simulink model "Solution3_RFReceiverWithXdipole"  (R2024b)
settings: Solver=VariableStepAuto  StartTime=0.0  StopTime=inf  RelTol=1e-3  EnableMultiTasking=on
PreLoadFcn:
  | % Baseband parameters
  | bitRate = 250e3;
  | spf = 4;  % samples per frame
  | bps = 4;  % bits per ZigBee symbol
  | sps = 16;  % samples per OQPSK symbol
  | cps = 32;  % chips per ZigBee symbol
  | chipRate = bitRate * cps / bps;
  | 
  | % RF parameters
  | carrierFreqs = [2.45 2.5]*1e9;  % Hz
  | harmonicOrder = [1 3];
  | oversampling = 4;  % reduce RF simulation step size to simulate interferer
  | load('XdipoleAntenna.mat')
undefined symbols (not defined in the file): rational, S, SampTime, sparameters
libraries: simrfV2elements x7, commdigbbndpm3 x3, simrfV2util1 x3, commrandsrc3 x2, dspmathops x2, dspsigops x2, dspstat3 x2, matrix_library x2, simulink x1, commrfcorlib x1, commrflib2 x1, commsink2 x1
Description:
  | Top-Down Design of Spread Spectrum Receiver for ZigBee
settings Model: Creator=The MathWorks, Inc.  LastModifiedBy=maxnolan
settings SolverCC: AlgebraicLoopSolver=TrustRegion  MinimalZcImpactIntegration=on  MaxZcPerStep=1
settings DataIOCC: LimitDataPoints=on  SaveFormat=Array  SaveOutput=off  SignalLogging=off  DSMLogging=off  SaveTime=off  ReturnWorkspaceOutputs=off
settings OptimizationCC: ReuseModelBlockBuffer=off  ExpressionDepthLimit=2147483647  LifeSpan=inf
settings DebuggingCC: ConsistencyChecking=warning  UnderspecifiedInitializationDetection=Classic  MergeDetectMultiDrivingBlocksExec=none  TimeAdjustmentMsg=warning  MaxConsecutiveZCsMsg=warning  SolverPrmCheckMsg=warning  FcnCallInpInsideContextMsg=warning  UnconnectedInputMsg=warning  UnconnectedOutputMsg=warning  UnconnectedLineMsg=warning  StateNameClashWarn=warning  SFUnexpectedBacktrackingDiag=warning  SFNoUnconditionalDefaultTransitionDiag=warning  SFExecutionAtInitializationDiag=none  ArithmeticOperatorsInVariantConditions=warning
settings HardwareCC: ProdBitPerPointer=32  ProdBitPerSizeT=32  ProdBitPerPtrDiffT=32  ProdLargestAtomicFloat=None  ProdIntDivRoundTo=Undefined  ProdEndianess=Unspecified  ProdWordSize=32  ProdHWDeviceType=32-bit Generic
settings ModelReferenceCC: EnableRefExpFcnMdlSchedulingChecks=on  PropagateSignalLabelsOutOfModel=off
settings SFSimCC: SimUseLocalCustomCode=off
settings RTWCC: RTWUseLocalCustomCode=off  BuildConfiguration=Faster Runs  GPUComputeCapability=3.5  DLArmComputeVersion=19.05
settings CodeAppCC: StateflowObjectComments=on
settings GRTTargetCC: TargetLangStandard=C89/C90 (ANSI)  CombineOutputUpdateFcns=off  GRTInterface=on
settings ConfigComp: CovMetricSettings=dw  CovSaveCumulativeToWorkspaceVar=on  CovSaveSingleToWorkspaceVar=on  CovExternalEMLEnable=off  CovSFcnEnable=off
settings SimscapeCC: SimscapeNormalizeSystem=off  SimscapeNominalValues="[{\"value\":\"10\",\"unit\":\"V\"},{\"value\":\"1\",\"unit\":\"A\"},{\"value\":\"10\",\"unit\":\"N*m\"},{\"value\":\"10\",\"unit\":\"bar\"},{\"value\":\"100\",\"unit\":\"kJ/kg\"},{\"value\":\"1\",\"unit\":\"kW\"},{\"value\":\"300\",\"unit\":\"K\"},{\"value\":\"100\",\"unit\":\"cm^3/s\"},{\"value\":\"1\",\"unit\":\"kN\"},{\"value\":\"1\",\"unit\":\"g/cm^3\"},{\"value\":\"1\",\"unit\":\"l\"},{\"value\":\"1\",\"unit\":\"cm^2\"},{\"value\":\"60\",\"unit\":\"Hz\"}]"
settings ConfigurationSet: Description=SimMechanics 2G

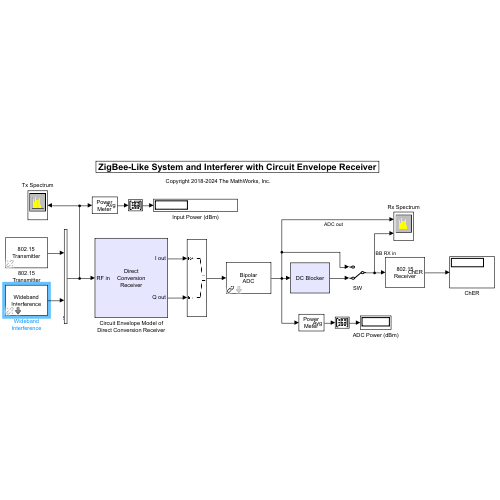
[thumbnail: Simulink's stored preview of the top-level diagram]
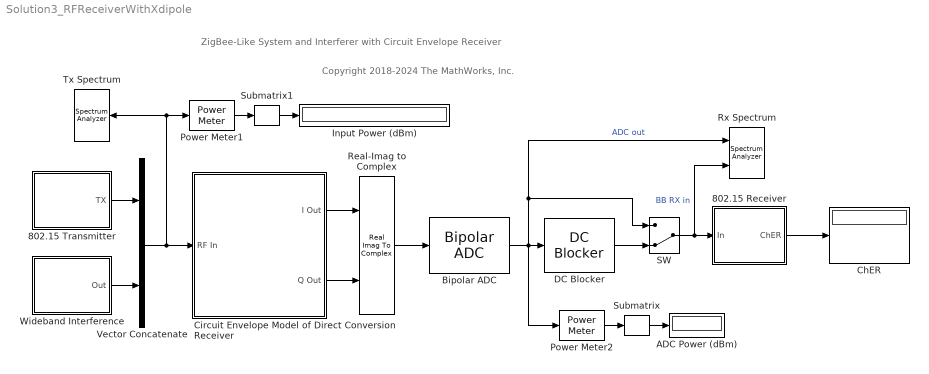
== system Solution3_RFReceiverWithXdipole ==
  note: ZigBee-Like System and Interferer with Circuit Envelope Receiver
  note: Copyright 2018-2024 The MathWorks, Inc.
  802.15 Transmitter : Subsystem  AncestorBlock=TopDownRFReceiverDesignLib/802.15 Transmitter
      mask Display: disp('802.15\nTransmitter')
  802.15 Receiver : Subsystem
      mask Display:
      | disp('802.15\nReceiver')
      | port_label('output', 1, 'ChER')
  ADC Power (dBm) : Display
  Bipolar ADC : TopDownRFReceiverDesignLib/Bipolar ADC  FS_V=sqrt(10^((0-30)/10))  N=10
      settings: LibrarySourceBlock=commdemoslib/Bipolar ADC
  ChER : Display
  Circuit Envelope Model of Direct Conversion Receiver : Subsystem
      mask Display:
      | disp('Direct\nConversion\nReceiver')
      | port_label('input', 1, 'RF in')
      | port_label('output', 1, 'I out')
      | port_label('output', 2, 'Q out')
  DC Blocker : dspsigops/DC Blocker  Algorithm=IIR  NormalizedBandwidth=0.001  Length=64  Order=16  SimulateUsing=Interpreted execution
  Input Power (dBm) : Display
  Power Meter1 : dspstat3/Power Meter  Measurement=Average power  ReferenceLoad=1  OutputPowerUnits=dBm  WindowLength=1024  OverlapLength=1023  AllowArbitraryInputLength=off  ComputeCCDF=off  PowerRange=50  PowerResolution=0.1  CCDFOutput=Relative power (dB above average power)  ProbabilityVector=[ 10; 1; 0.1; 0.01; 0.001; 0.0001 ]  RelativePowerVector=[ 0; 3; 6; 9; 12 ]  ResetPort=off  SimulateUsing=Code generation
      settings: LibrarySourceBlock=commutil2/Power Meter
  Power Meter2 : dspstat3/Power Meter  Measurement=Average power  ReferenceLoad=1  OutputPowerUnits=dBm  WindowLength=1024  OverlapLength=1023  AllowArbitraryInputLength=off  ComputeCCDF=off  PowerRange=50  PowerResolution=0.1  CCDFOutput=Relative power (dB above average power)  ProbabilityVector=[ 10; 1; 0.1; 0.01; 0.001; 0.0001 ]  RelativePowerVector=[ 0; 3; 6; 9; 12 ]  ResetPort=off  SimulateUsing=Code generation
      settings: LibrarySourceBlock=commutil2/Power Meter
  Real-Imag to Complex : RealImagToComplex
  Rx Spectrum : SpectrumAnalyzer  NumInputPorts=2  WindowPosition=[540.000000,122.000000,475.000000,318.000000,]  ScopeFrameLocation=window  Method=Welch  SampleRate=16000000  AxesScaling=Manual  FrequencyResolutionMethod=Window length  RBWSource=Property  RBW=46921.92192  FFTLength=128  Span=32000000  StartFrequency=-16000000  StopFrequency=16000000  AveragingMethod=Running  SpectralAverages=16  YLabel=Power  YLimits=[-75.64216798,-32.23249525]  ShowLegend=on  AllowFFTLengthLessThanSamplesPerUpdate=on  SegLen=1024
  SW : ManualSwitch  CurrentSetting=0
  Submatrix : matrix_library/Submatrix  RowSpan=One row  RowStartMode=Last  RowStartIndex=1  RowEndMode=Last  RowEndIndex=1  ColSpan=One column  ColStartMode=Last  ColStartIndex=1  ColEndMode=Last  ColEndIndex=1
  Submatrix1 : matrix_library/Submatrix  RowSpan=One row  RowStartMode=Last  RowStartIndex=1  RowEndMode=Last  RowEndIndex=1  ColSpan=Range of columns  ColStartMode=Offset from last  ColStartIndex=1  ColEndMode=Last  ColEndIndex=1
  Tx Spectrum : SpectrumAnalyzer  WindowPosition=[21.000000,122.000000,520.000000,320.000000,]  ScopeFrameLocation=window  Method=Welch  SampleRate=16000000  AxesScaling=Manual  FrequencyResolutionMethod=Window length  RBWSource=Property  RBW=46921.92192  FFTLength=128  Span=16000000  StartFrequency=-16000000  StopFrequency=16000000  AveragingMethod=Running  SpectralAverages=16  FrequencyOffset=carrierFreqs  YLabel=Power  YLimits=[-211.4024859,-30.13598267]  ShowLegend=on  AllowFFTLengthLessThanSamplesPerUpdate=on  SegLen=1024
  Vector Concatenate : Concatenate  Mode=Multidimensional array  ConcatenateDimension=2
  Wideband Interference : Subsystem  AncestorBlock=TopDownRFReceiverDesignLib/Wideband Interference  mask{Pout=-30}
      mask prompts: Pout "Output power (dBm)"
      mask Display: disp('Wideband\nInterference')
  wires:
  802.15 Receiver/1(ChER) -> ChER/1
  Circuit Envelope Model of Direct Conversion Receiver/1(I Out) -> Real-Imag to Complex/1
  Circuit Envelope Model of Direct Conversion Receiver/2(Q Out) -> Real-Imag to Complex/2
  Bipolar ADC/1 -> Power Meter2/1, DC Blocker/1, SW/1, Rx Spectrum/1  "ADC out"
  Vector Concatenate/1 -> Circuit Envelope Model of Direct Conversion Receiver/1(RF In), Tx Spectrum/1, Power Meter1/1
  Power Meter1/1 -> Submatrix1/1
  802.15 Transmitter/1(TX) -> Vector Concatenate/1
  Power Meter2/1 -> Submatrix/1
  DC Blocker/1 -> SW/2
  SW/1 -> Rx Spectrum/2, 802.15 Receiver/1(In)  "BB RX in"
  Submatrix/1 -> ADC Power (dBm)/1
  Submatrix1/1 -> Input Power (dBm)/1
  Wideband Interference/1(Out) -> Vector Concatenate/2
  Real-Imag to Complex/1 -> Bipolar ADC/1

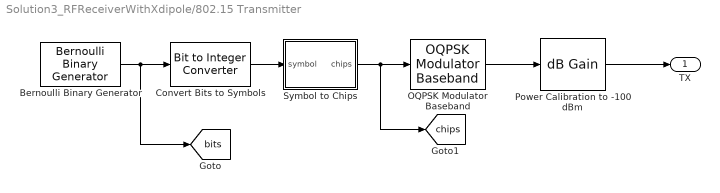
== system Solution3_RFReceiverWithXdipole/802.15 Transmitter ==
  Bernoulli Binary Generator : commrandsrc3/Bernoulli Binary Generator  ProbabilityOfZero=0.5  SeedSource=Parameter  Seed=73  SampleTime=1/bitRate  SamplesPerFrame=spf  OutputDataType=double  SimulateUsing=Interpreted execution
  Convert Bits to Symbols : simulink/Logic and Bit Operations/Bit to Integer Converter  nbits=4  bitOrder=MSB first  signedOutputValues=Unsigned  outDtype=Inherit via internal rule  outDtypeSigned=Inherit via internal rule
      settings: LibrarySourceBlock=|
      | commutil2/Bit to Integer
      | Converter
  OQPSK Modulator Baseband : commdigbbndpm3/OQPSK Modulator Baseband  InType=Bit  Ph=0  Mapping=Gray  pulseShape=Half sine  num=[0.7071, 0.7071]  rolloff=0.2  filterSpan=10  sps=sps  RateOptions=Enforce single-rate processing  outDtype=double
  Power Calibration to -100 dBm : dspmathops/dB Gain  dB="-130  % power of preceding block is 1 W"  intype=Amplitude
  Symbol to Chips : MATLAB Function  TreatAsAtomicUnit=on
  TX : Outport  VectorParamsAs1DForOutWhenUnconnected=off
  tag scope: bits=global, chips=global
  wires:
  Bernoulli Binary Generator/1 -> [bits], Convert Bits to Symbols/1
  Symbol to Chips/1(chips) -> [chips], OQPSK Modulator Baseband/1
  Convert Bits to Symbols/1 -> Symbol to Chips/1(symbol)
  OQPSK Modulator Baseband/1 -> Power Calibration to -100 dBm/1
  Power Calibration to -100 dBm/1 -> TX/1

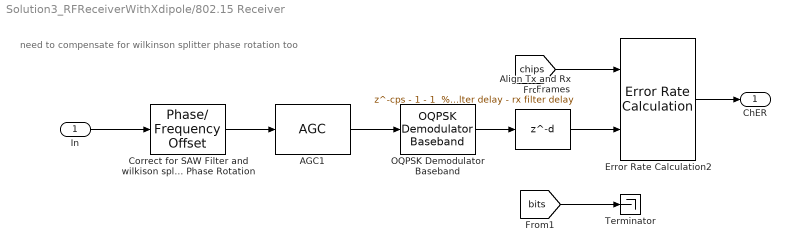
== system Solution3_RFReceiverWithXdipole/802.15 Receiver ==
  note: need to compensate for wilkinson splitter phase rotation too
  In : Inport
  AGC1 : commrfcorlib/AGC  LegacyMode=off  DetectorMethod=Rectifier  LoopMethod=Linear  UpdatePeriod=100  StepSize=0.1  AdaptationStepSize=0.01  DesiredOutputPower=1  AveragingLength=100  MaximumGain=30  MaxPowerGain=200  GainOutputPort=off  InputPowerOutputPort=off  SimulateUsing=Interpreted execution
  Align Tx and Rx Frames : Delay  DelayLength="cps - 1 - 1  % chips/sym - tx filter delay - rx filter delay"  InputProcessing=Columns as channels (frame based)
  Correct for SAW Filter and wilkison splitter Phase Rotation : commrflib2/Phase// Frequency Offset  phaseOffset=115-90  freqPort=off  freqOffset=0
  Error Rate Calculation2 : commsink2/Error Rate Calculation  N="32  % 1 frame of chips"  st_delay=2e3  cp_mode=Entire frame  subframe=[]  PMode=Port  WsName=ErrorVec  RsMode2=off  stop=on  numErr=1e3  maxBits=1e7
  OQPSK Demodulator Baseband : commdigbbndpm3/OQPSK Demodulator Baseband  OutType=Bit  Ph=0  Mapping=Gray  pulseShape=Half sine  num=[0.7071, 0.7071]  rolloff=0.2  filterSpan=10  sps=sps  RateOptions=Enforce single-rate processing  outDtype2=double
  Terminator : Terminator
  ChER : Outport  VectorParamsAs1DForOutWhenUnconnected=off
  wires:
  Correct for SAW Filter and wilkison splitter Phase Rotation/1 -> AGC1/1
  Error Rate Calculation2/1 -> ChER/1
  [chips] -> Error Rate Calculation2/1
  In/1 -> Correct for SAW Filter and wilkison splitter Phase Rotation/1
  Align Tx and Rx Frames/1 -> Error Rate Calculation2/2
  OQPSK Demodulator Baseband/1 -> Align Tx and Rx Frames/1
  AGC1/1 -> OQPSK Demodulator Baseband/1
  [bits] -> Terminator/1

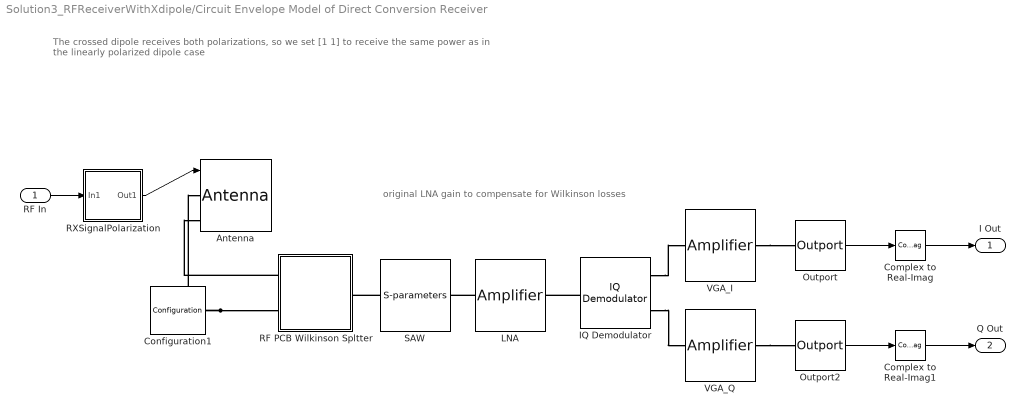
== system Solution3_RFReceiverWithXdipole/Circuit Envelope Model of Direct Conversion Receiver ==
  note: The crossed dipole receives both polarizations,
      | so we set [1 1] to receive the same power as in the linearly polarized dipole case
  note: original LNA gain to compensate for Wilkinson losses
  RF In : Inport
  Antenna : simrfV2elements/Antenna  CacheLevel=0  AntennaSource=Antenna object  PrevAppliedAntSource=Antenna object  Gr=0 dBi  Zin=50  AntennaObj=Xdipole  InputIncWave=on  OutputRadWave=off  CarrierFreqInc=carrierFreqs Hz  rArr=[0 0] deg  CarrierFreqRad=2.1 GHz  rDep=[0 0] deg  AddNoise=on  InternalGrounding=on  SparamRepresentationImp=Time domain  FitTolImp=-40  AutoImpulseLengthImp=on  ImpulseLengthImp=1e-10 s
  Complex to Real-Imag : ComplexToRealImag  Output=Real
  Complex to Real-Imag1 : ComplexToRealImag  Output=Real
  Configuration1 : simrfV2util1/Configuration  AutoFreq=off  Tones=carrierFreqs Hz  Harmonics=harmonicOrder  NormalizeCarrierPower=on  SolverType=Auto  UseCCode=on  StepSize=1/(2*chipRate*oversampling) s  AddNoise=on  defaultRNG=off  Seed=0  Temperature=290.0 K  SolverDelFlag=0  AbsTol=1e-6  RelTol=1e-3  MaxIter=10  ErrorEstimationType=2-norm over all variables  EnableInterpFilter=off  HiddenFIRfilterControllerParam=off  SmallSignalApprox=off  AllSimFreqs=on  SimFreqs=[] Hz  SimFreqsInternal=[]  SamplesPerFrame=cps * sps / 2
  "IQ Demodulator " : simrfV2systems/IQ Demodulator  classname=iqdemod  Source_linear_gain=Available power gain  linear_gain=-7 dB  Poly_Coeffs=[0 1]  LOFreq=2.45e9 Hz  Zin=50  Zout=50  AddIRFilter=off  AddCSFilters=on  InternalGrounding=on  ForceNextInit=off  Source_Poly=Even and odd order  IPType=Input  IP2=55 dBm  IP3=inf dBm  P1dB=inf dBm  Psat=inf dBm  Gcomp=inf dBm  NF=10  GainMismatch=0 dB  PhaseMismatch=0 deg  Isolation=105 dB  AddPhaseNoise=on  PhaseNoiseOffset=[0.2 1 2 3 7]*1e6  PhaseNoiseLevel=[-70 -80 -95 -110 -120]  AutoImpulseLengthPN=on  ImpulseLengthPN=5e-6  ImpulseLength_unitPN=s  DesignMethodIR=Ideal  ResponseTypeIR=Highpass  ImplementationIR=LC Tee  ImplementationIdealIR=Constant per carrier  ImplementationRationalIR=Transfer function  UseFilterOrderIR=on  FilterOrderIR=3  PassFreq_lpIR=1  PassFreq_lp_unitIR=GHz  PassFreq_hpIR=2  PassFreq_hp_unitIR=GHz  PassFreq_bpIR=[2 3]  PassFreq_bp_unitIR=GHz  PassFreq_bsIR=[1 4]  PassFreq_bs_unitIR=GHz  PassAttenIR=10*log10(2)  StopFreq_lpIR=2  StopFreq_lp_unitIR=GHz  StopFreq_hpIR=1  StopFreq_hp_unitIR=GHz  StopFreq_bpIR=[1.5 3.5]  StopFreq_bp_unitIR=GHz  StopFreq_bsIR=[2.1 2.9]  StopFreq_bs_unitIR=GHz  StopAttenIR=40  RsrcIR=50  RloadIR=50  AutoImpulseLengthIR=on  ImpulseLengthIR=1e-10  ImpulseLength_unitIR=s  DesignMethodCS=Ideal  ResponseTypeCS=Lowpass  ImplementationCS=LC Tee  ImplementationIdealCS=Constant per carrier  ImplementationRationalCS=Transfer function  UseFilterOrderCS=on  FilterOrderCS=3  PassFreq_lpCS=50  PassFreq_lp_unitCS=MHz  PassFreq_hpCS=2  PassFreq_hp_unitCS=GHz  PassFreq_bpCS=[2 3]  PassFreq_bp_unitCS=GHz  PassFreq_bsCS=[1 4]  PassFreq_bs_unitCS=GHz  PassAttenCS=10*log10(2)  StopFreq_lpCS=2  StopFreq_lp_unitCS=GHz  StopFreq_hpCS=1  StopFreq_hp_unitCS=GHz  StopFreq_bpCS=[1.5 3.5]  StopFreq_bp_unitCS=GHz  StopFreq_bsCS=[2.1 2.9]  StopFreq_bs_unitCS=GHz  StopAttenCS=40  RsrcCS=50  RloadCS=50  AutoImpulseLengthCS=on  ImpulseLengthCS=1e-10  ImpulseLength_unitCS=s
  LNA : simrfV2elements/Amplifier  classname=amplifier  DataSource=Data file  File=unitygain.s2p  isNetworkObj=off  NetworkObject=sparameters('default.s2p')  Paramtype=S-parameters  Sparam=[0 0;1 0]  SparamFreq=1e9 Hz  SparamZ0=50  isRationalObj=off  RationalObject=rational('default.s2p')  Residues=0  Poles=0  DF={0 0; 1 0}  Source_linear_gain=Available power gain  linear_gain=22 dB  AmAmAmPmTable=[-25,5,-1;-10,20,-2;0,27,5;5,28,12]  Zin=50  Zout=50  Source_Poly=Even and odd order  Poly_Coeffs=[0 1]  IPType=Output  IP2=Inf dBm  IP3=30 dBm  P1dB=inf dBm  Psat=inf dBm  Gcomp=inf dBm  InternalGrounding=on  SourceFreq=Extracted from data source  PlotFreq=[1e9:1e6:3e9] Hz  PlotType=X-Y plane  YParam1=S(1,1)  YFormat1=Magnitude (dB)  YParam2=None  YFormat2=Magnitude (dB)  YOption=Linear  XOption=Linear  SparamRepresentation=Time domain  FitTol=-40  FitOpt=Fit individually  MaxPoles=48  AutoImpulseLength=on  ImpulseLength=1e-10 s  MagModeling=off  AddNoise=on  NoiseType=Noise figure  NoiseDist=White  NF=7  MinNF=0  Gopt=0  RN=0  CarrierFreq=0 Hz  NoiseAutoImpulseLength=on  NoiseImpulseLength=1e-10 s  ConstS21NL=on  OpFreq=0 Hz  SetOpFreqAsMaxS21=on
  Outport : simrfV2util1/Outport  SensorType=Power  OutputFormat=Complex Baseband  CarrierFreq=0 Hz  ZL=50  InternalGrounding=on  StepSize=1e-6 s  AutoStep=on  HalfPolyphaseLength=0
  Outport2 : simrfV2util1/Outport  SensorType=Power  OutputFormat=Complex Baseband  CarrierFreq=0 Hz  ZL=50  InternalGrounding=on  StepSize=1e-6 s  AutoStep=on  HalfPolyphaseLength=0
  RF PCB Wilkinson Spltter : Subsystem
  RXSignalPolarization : Subsystem  mask{pol1=[1 1], pol2=[1 1]}
      mask prompts: pol1 "Polarization Signal [V H]"; pol2 "Polarization Interferer [V H]"
      mask init:
      | Pol = ones(256,2,2);
      | Pol(:,1,1) = pol1(1)/sqrt(sum(pol1));
      | Pol(:,1,2) = pol1(2)/sqrt(sum(pol1));
      | Pol(:,2,1) = pol2(1)/sqrt(sum(pol2));
      | Pol(:,2,2) = pol2(2)/sqrt(sum(pol2));
      mask DialogControl DescGroupVar Prompt: Signal polarization
      mask DialogControl DescTextVar Prompt: Set the polarization of the input signals with an array representing the amount of power on the V and H components respecitvely. This block preserves the input power.
  SAW : simrfV2elements/S-parameters  classname=sparam_element  DataSource=Data file  File=SAWfilter.s2p  isNetworkObj=off  NetworkObject=sparameters('default.s2p')  Paramtype=S-parameters  Sparam=[0 0;1 0]  SparamFreq=1e9 Hz  SparamZ0=50  isRationalObj=off  RationalObject=rational('default.s2p')  Residues=0  Poles=0  DF={0 0; 1 0}  FitOpt=Fit individually  FitTol=-30  MaxPoles=48  SourceFreq=Extracted from data source  PlotFreq=[1e9:1e6:3e9] Hz  PlotType=X-Y plane  YParam1=S(2,1)  YFormat1=Angle (degrees)  YParam2=None  YFormat2=Magnitude (dB)  YOption=Linear  XOption=Linear  AddNoise=on  InternalGrounding=on  SparamRepresentation=Time domain  AutoImpulseLength=off  ImpulseLength=SampTime*256 s  MagModeling=off  CacheLevel=0
  VGA_I : simrfV2elements/Amplifier  classname=amplifier  DataSource=Data file  File=unitygain.s2p  isNetworkObj=off  NetworkObject=sparameters('default.s2p')  Paramtype=S-parameters  Sparam=[0 0;1 0]  SparamFreq=1e9 Hz  SparamZ0=50  isRationalObj=off  RationalObject=rational('default.s2p')  Residues=0  Poles=0  DF={0 0; 1 0}  Source_linear_gain=Available power gain  linear_gain=40 dB  AmAmAmPmTable=[-25,5,-1;-10,20,-2;0,27,5;5,28,12]  Zin=50  Zout=50  Source_Poly=Even and odd order  Poly_Coeffs=[0 1]  IPType=Output  IP2=Inf dBm  IP3=35 dBm  P1dB=inf dBm  Psat=inf dBm  Gcomp=inf dBm  InternalGrounding=on  SourceFreq=Extracted from data source  PlotFreq=[1e9:1e6:3e9] Hz  PlotType=X-Y plane  YParam1=S(1,1)  YFormat1=Magnitude (dB)  YParam2=None  YFormat2=Magnitude (dB)  YOption=Linear  XOption=Linear  SparamRepresentation=Time domain  FitTol=-40  FitOpt=Fit individually  MaxPoles=48  AutoImpulseLength=on  ImpulseLength=1e-10 s  MagModeling=off  AddNoise=on  NoiseType=Noise figure  NoiseDist=White  NF=14  MinNF=0  Gopt=0  RN=0  CarrierFreq=0 Hz  NoiseAutoImpulseLength=on  NoiseImpulseLength=1e-10 s  ConstS21NL=on  OpFreq=0 Hz  SetOpFreqAsMaxS21=on
  VGA_Q : simrfV2elements/Amplifier  classname=amplifier  DataSource=Data file  File=unitygain.s2p  isNetworkObj=off  NetworkObject=sparameters('default.s2p')  Paramtype=S-parameters  Sparam=[0 0;1 0]  SparamFreq=1e9 Hz  SparamZ0=50  isRationalObj=off  RationalObject=rational('default.s2p')  Residues=0  Poles=0  DF={0 0; 1 0}  Source_linear_gain=Available power gain  linear_gain=40 dB  AmAmAmPmTable=[-25,5,-1;-10,20,-2;0,27,5;5,28,12]  Zin=50  Zout=50  Source_Poly=Even and odd order  Poly_Coeffs=[0 1]  IPType=Output  IP2=Inf dBm  IP3=35 dBm  P1dB=inf dBm  Psat=inf dBm  Gcomp=inf dBm  InternalGrounding=on  SourceFreq=Extracted from data source  PlotFreq=[1e9:1e6:3e9] Hz  PlotType=X-Y plane  YParam1=S(1,1)  YFormat1=Magnitude (dB)  YParam2=None  YFormat2=Magnitude (dB)  YOption=Linear  XOption=Linear  SparamRepresentation=Time domain  FitTol=-40  FitOpt=Fit individually  MaxPoles=48  AutoImpulseLength=on  ImpulseLength=1e-10 s  MagModeling=off  AddNoise=on  NoiseType=Noise figure  NoiseDist=White  NF=14  MinNF=0  Gopt=0  RN=0  CarrierFreq=0 Hz  NoiseAutoImpulseLength=on  NoiseImpulseLength=1e-10 s  ConstS21NL=on  OpFreq=0 Hz  SetOpFreqAsMaxS21=on
  I Out : Outport  VectorParamsAs1DForOutWhenUnconnected=off
  Q Out : Outport  Port=2  VectorParamsAs1DForOutWhenUnconnected=off
  wires:
  Complex to Real-Imag1/1 -> Q Out/1
  Outport2/1 -> Complex to Real-Imag1/1
  Complex to Real-Imag/1 -> I Out/1
  Outport/1 -> Complex to Real-Imag/1
  RF In/1 -> RXSignalPolarization/1(In1)
  RXSignalPolarization/1(Out1) -> Antenna/1
  connections:
  Configuration1/LConn1 -- RF PCB Wilkinson Spltter/RConn2 -- Antenna/LConn1
  VGA_I/RConn1 -- Outport/LConn1
  VGA_Q/RConn1 -- Outport2/LConn1
  LNA/LConn1 -- SAW/RConn1
  "IQ Demodulator "/RConn1 -- VGA_I/LConn1
  "IQ Demodulator "/LConn1 -- LNA/RConn1
  "IQ Demodulator "/RConn2 -- VGA_Q/LConn1
  SAW/LConn1 -- RF PCB Wilkinson Spltter/LConn1
  RF PCB Wilkinson Spltter/RConn1 -- Antenna/LConn2

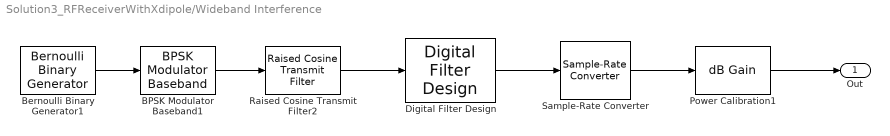
== system Solution3_RFReceiverWithXdipole/Wideband Interference ==
  BPSK Modulator Baseband1 : commdigbbndpm3/BPSK Modulator Baseband  Ph=0  outDtype=double  outWordLen=16  outUDDataType=sfix(16)  outFracLenMode=Best precision  outFracLen=15  outDataTypeStr=double  outLastDataTypeStr=double
  Bernoulli Binary Generator1 : commrandsrc3/Bernoulli Binary Generator  ProbabilityOfZero=0.5  SeedSource=Parameter  Seed=612  SampleTime="1/4e6  % 1/3.846e6"  SamplesPerFrame="640  % 1923"  OutputDataType=double  SimulateUsing=Interpreted execution
  Digital Filter Design : dspfdesign/Digital Filter Design  mwdsp_browser_bugfix_var=off
  Power Calibration1 : dspmathops/dB Gain  dB=10.2-30+Pout  intype=Amplitude
  Raised Cosine Transmit Filter2 : commfilt2/Raised Cosine Transmit Filter  filtType=Square root  R=0.2  filtSpan=10  N=10  filterGain=1  InputProcessing=Columns as channels (frame based)  RateOptions=Allow multirate processing  framing=Mute  checkCoeff=off  variableName=rcTxFilt2  checkGain=Normalized  sampMode=Mute  saveAsFlag=0  currentFiltSpan=10  D=(10)/2  launchFVT=on  roundingMode=Floor  overflowMode=off  coeffDataTypeStr=Inherit: Same word length as input  coeffMin=[]  coeffMax=[]  coeffLastDataTypeStr=Inherit: Same word length as input  outputDataTypeStr=Inherit: Same as accumulator  outputMin=[]  outputMax=[]  outputLastDataTypeStr=Inherit: Same as accumulator
  Sample-Rate Converter : dspsigops/Sample-Rate Converter  InputSampleRate="40e6  % 38.46e6"  OutputSampleRate=2*chipRate*oversampling  OutputRateTolerance=0  Bandwidth="2*4  % 2*3.846"  StopbandAttenuation=60  AllowArbitraryInputLength=off  SimulateUsing=Interpreted execution
  Out : Outport  VectorParamsAs1DForOutWhenUnconnected=off
  wires:
  Digital Filter Design/1 -> Sample-Rate Converter/1
  BPSK Modulator Baseband1/1 -> Raised Cosine Transmit Filter2/1
  Bernoulli Binary Generator1/1 -> BPSK Modulator Baseband1/1
  Raised Cosine Transmit Filter2/1 -> Digital Filter Design/1
  Sample-Rate Converter/1 -> Power Calibration1/1
  Power Calibration1/1 -> Out/1

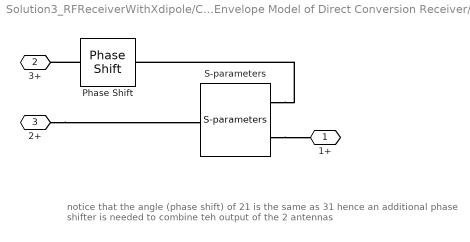
== system Solution3_RFReceiverWithXdipole/Circuit Envelope Model of Direct Conversion Receiver/RF PCB Wilkinson Spltter ==
  note: notice that the angle (phase shift) of 21 is the same as 31
      | hence an additional phase shifter is needed to combine teh output of the 2 antennas
  Phase Shift : simrfV2elements/Phase Shift  PhaseShift=-90 deg  InternalGrounding=on
  S-parameters : simrfV2elements/S-parameters  classname=sparam_element  DataSource=Data file  File=wilkinsonSplitterSparams.s3p  isNetworkObj=on  NetworkObject=sWilk  Paramtype=S-parameters  Sparam=[0 0;1 0]  SparamFreq=1e9 Hz  SparamZ0=50  isRationalObj=off  RationalObject=rational('default.s2p')  Residues=0  Poles=0  DF={0 0; 1 0}  FitOpt=Share all poles  FitTol=-40  MaxPoles=48  SourceFreq=Extracted from data source  PlotFreq=[1e9:1e6:3e9] Hz  PlotType=X-Y plane  YParam1=S(2,1)  YFormat1=Angle (degrees)  YParam2=None  YFormat2=Angle (degrees)  YOption=Linear  XOption=Linear  AddNoise=on  InternalGrounding=on  SparamRepresentation=Time domain  AutoImpulseLength=on  ImpulseLength=1e-10 s  MagModeling=off  CacheLevel=0
  1+ : PMIOPort  Side=Left
  3+ : PMIOPort  Port=2  Side=Right
  2+ : PMIOPort  Port=3  Side=Right
  connections:
  S-parameters/LConn2 -- Phase Shift/RConn1
  S-parameters/LConn1 -- 1+/RConn1
  2+/RConn1 -- S-parameters/RConn1
  Phase Shift/LConn1 -- 3+/RConn1

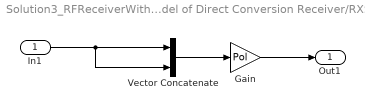
== system Solution3_RFReceiverWithXdipole/Circuit Envelope Model of Direct Conversion Receiver/RXSignalPolarization ==
  In1 : Inport
  Gain : Gain  Gain=Pol
  Vector Concatenate : Concatenate  Mode=Multidimensional array  ConcatenateDimension=3
  Out1 : Outport
  wires:
  In1/1 -> Vector Concatenate/2, Vector Concatenate/1
  Vector Concatenate/1 -> Gain/1
  Gain/1 -> Out1/1

== matlab function Solution3_RFReceiverWithXdipole/802.15 Transmitter/Symbol to Chips ==
  data: symbol input; chips output size=[32 1]
function chips = sym2chips(symbol)
  chipMap = ...
     [1 1 0 1 1 0 0 1 1 1 0 0 0 0 1 1 0 1 0 1 0 0 1 0 0 0 1 0 1 1 1 0;
      1 1 1 0 1 1 0 1 1 0 0 1 1 1 0 0 0 0 1 1 0 1 0 1 0 0 1 0 0 0 1 0;
      0 0 1 0 1 1 1 0 1 1 0 1 1 0 0 1 1 1 0 0 0 0 1 1 0 1 0 1 0 0 1 0;
      0 0 1 0 0 0 1 0 1 1 1 0 1 1 0 1 1 0 0 1 1 1 0 0 0 0 1 1 0 1 0 1;
      0 1 0 1 0 0 1 0 0 0 1 0 1 1 1 0 1 1 0 1 1 0 0 1 1 1 0 0 0 0 1 1;
      0 0 1 1 0 1 0 1 0 0 1 0 0 0 1 0 1 1 1 0 1 1 0 1 1 0 0 1 1 1 0 0;
      1 1 0 0 0 0 1 1 0 1 0 1 0 0 1 0 0 0 1 0 1 1 1 0 1 1 0 1 1 0 0 1;
      1 0 0 1 1 1 0 0 0 0 1 1 0 1 0 1 0 0 1 0 0 0 1 0 1 1 1 0 1 1 0 1;
      1 0 0 0 1 1 0 0 1 0 0 1 0 1 1 0 0 0 0 0 0 1 1 1 0 1 1 1 1 0 1 1;
      1 0 1 1 1 0 0 0 1 1 0 0 1 0 0 1 0 1 1 0 0 0 0 0 0 1 1 1 0 1 1 1;
      0 1 1 1 1 0 1 1 1 0 0 0 1 1 0 0 1 0 0 1 0 1 1 0 0 0 0 0 0 1 1 1;
      0 1 1 1 0 1 1 1 1 0 1 1 1 0 0 0 1 1 0 0 1 0 0 1 0 1 1 0 0 0 0 0;
      0 0 0 0 0 1 1 1 0 1 1 1 1 0 1 1 1 0 0 0 1 1 0 0 1 0 0 1 0 1 1 0;
      0 1 1 0 0 0 0 0 0 1 1 1 0 1 1 1 1 0 1 1 1 0 0 0 1 1 0 0 1 0 0 1;
      1 0 0 1 0 1 1 0 0 0 0 0 0 1 1 1 0 1 1 1 1 0 1 1 1 0 0 0 1 1 0 0;
      1 1 0 0 1 0 0 1 0 1 1 0 0 0 0 0 0 1 1 1 0 1 1 1 1 0 1 1 1 0 0 0];

 chips = chipMap(1+symbol,:)'; % +1 for 1-based indexing
